simulink model "simulink_CartpendDiscrete_KControl"  (R2017b)
settings: Solver=ode45  StartTime=0.0  StopTime=10  MaxStep=0.01  RelTol=1e-3  EnableMultiTasking=on
undefined symbols (not defined in the file): bT, bX, distThetaAccVariance, distXAccVariance, g, K, L, mc, mp, sensorNoiseVariance, tSamp, y0, yGoal
settings Model: Creator=Thomas  LastModifiedBy=Thomas
settings DataIOCC: ExternalInput=t  InitialState=yIn  LimitDataPoints=on  SaveFormat=Array  SaveState=on
settings OptimizationCC: LifeSpan=inf
settings DebuggingCC: SFUnexpectedBacktrackingDiag=warning  SFNoUnconditionalDefaultTransitionDiag=warning  SFExecutionAtInitializationDiag=none
settings HardwareCC: ProdBitPerPointer=32  ProdBitPerSizeT=32  ProdBitPerPtrDiffT=32  ProdLargestAtomicFloat=None  ProdIntDivRoundTo=Undefined  ProdEndianess=Unspecified  ProdWordSize=32  ProdHWDeviceType=32-bit Generic
settings ModelReferenceCC: PropagateSignalLabelsOutOfModel=off
settings CodeAppCC: StateflowObjectComments=on
settings GRTTargetCC: TargetLangStandard=C89/C90 (ANSI)  GeneratePreprocessorConditionals=Disable all
settings ConfigComp: CovMetricSettings=dw  CovHtmlReporting=on  CovSaveCumulativeToWorkspaceVar=on  CovSaveSingleToWorkspaceVar=on  CovExternalEMLEnable=off

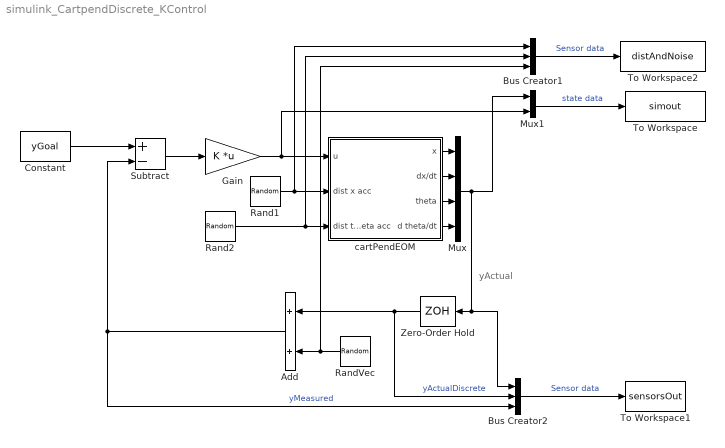
== system simulink_CartpendDiscrete_KControl ==
  note: yActual
  Add : Sum
  Bus Creator1 : BusCreator  Inputs=3
  Bus Creator2 : BusCreator  Inputs=3
  Constant : Constant  Value=yGoal  VectorParams1D=off
  Gain : Gain  Gain=K  Multiplication=Matrix(K*u) (u vector)
  Mux : Mux
  Mux1 : Mux  Inputs=2
  Rand1 : RandomNumber  Variance=distXAccVariance  Seed=4  SampleTime=tSamp
  Rand2 : RandomNumber  Variance=distThetaAccVariance  Seed=5  SampleTime=tSamp
  RandVec : RandomNumber  Variance=sensorNoiseVariance  Seed=[0,1,2,3]  SampleTime=tSamp
  Subtract : Sum  Inputs=+-
  To Workspace : ToWorkspace  VariableName=simout  SaveFormat=Structure With Time  SampleTime=-1
  To Workspace1 : ToWorkspace  VariableName=sensorsOut  SaveFormat=Timeseries  SampleTime=-1
  To Workspace2 : ToWorkspace  VariableName=distAndNoise  SaveFormat=Timeseries  SampleTime=-1
  Zero-Order Hold : ZeroOrderHold  SampleTime=tSamp
  cartPendEOM : Subsystem  mask(Inverted pendulum on cart){mc=mc, mp=mp, L=L, g=g, bX=bX, bT=bT}
      mask prompts: mc "Mass of cart (kg):"; mp "Mass of pendulum (kg):"; L "Distance to pendulum center of mass(m):"; g "Acceleration of gravity (m/s^2):"; bX "Damping of cart (kg/s)"; bT "Damping of pendulum (kg*m/s)"
      mask help: Unmask and double-click to see dynamics
      mask Help: Nonlinear dynamics of inverted pendulum on cart.
  wires:
  cartPendEOM/4(d theta/dt) -> Mux/4
  cartPendEOM/3("theta ") -> Mux/3
  cartPendEOM/2(dx/dt) -> Mux/2
  cartPendEOM/1(x) -> Mux/1
  Constant/1 -> Subtract/1
  Subtract/1 -> Gain/1
  Add/1 -> Bus Creator2/3, Subtract/2  "yMeasured"
  Bus Creator2/1 -> To Workspace1/1  "Sensor data"
  Mux1/1 -> To Workspace/1  "state data"
  Mux/1 -> Mux1/1, Bus Creator2/1, Zero-Order Hold/1
  Zero-Order Hold/1 -> Bus Creator2/2, Add/1  "yActualDiscrete"
  Gain/1 -> cartPendEOM/1(u), Mux1/2
  Rand1/1 -> Bus Creator1/1, cartPendEOM/2(dist x acc)
  Rand2/1 -> Bus Creator1/2, cartPendEOM/3("dist theta acc ")
  Bus Creator1/1 -> To Workspace2/1  "Sensor data"
  RandVec/1 -> Add/2, Bus Creator1/3

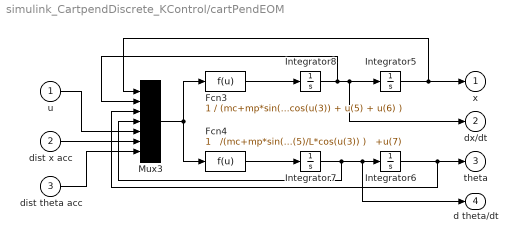
== system simulink_CartpendDiscrete_KControl/cartPendEOM ==
  u : Inport
  dist x acc : Inport  Port=2
  "dist theta acc " : Inport  Port=3
  Fcn3 : Fcn  Expr="1 / (mc+mp*sin(u(3))^2)  * (   u(4)^2*mp*L*sin(u(3)) -u(4)*bT/L*cos(u(3))   -u(2)*bX  -   mp*g*sin(u(3))*cos(u(3)) + u(5) + u(6) )"
  Fcn4 : Fcn  Expr="1   /(mc+mp*sin(u(3))^2)  * (   u(2)*bX/L*cos(u(3))   -   u(4)^2*mp*sin(u(3))*cos(u(3))   - u(4)*bT*(mc+mp)/ (L^2*mp)       + (mc+mp)*g/L*sin(u(3)) - u(5)/L*cos(u(3)) )   +u(7)"
  Integrator5 : Integrator  InitialCondition=y0(1)  ContinuousStateAttributes='x'
  Integrator6 : Integrator  InitialCondition=y0(3)  ContinuousStateAttributes='theta'
  Integrator7 : Integrator  InitialCondition=y0(4)  ContinuousStateAttributes='theta_dot'
  Integrator8 : Integrator  InitialCondition=y0(2)  ContinuousStateAttributes='xDot'
  Mux3 : Mux  Inputs=7
  x : Outport  InitialOutput=0
  dx/dt : Outport  Port=2  InitialOutput=0
  "theta " : Outport  Port=3  InitialOutput=0
  d theta/dt : Outport  Port=4  InitialOutput=0
  wires:
  Integrator5/1 -> Mux3/1, x/1
  Fcn4/1 -> Integrator7/1
  Mux3/1 -> Fcn3/1, Fcn4/1
  Fcn3/1 -> Integrator8/1
  Integrator8/1 -> Mux3/2, dx/dt/1, Integrator5/1
  Integrator7/1 -> Mux3/4, d theta/dt/1, Integrator6/1
  Integrator6/1 -> Mux3/3, "theta "/1
  u/1 -> Mux3/5
  dist x acc/1 -> Mux3/6
  "dist theta acc "/1 -> Mux3/7
